simulink model "SF023A_TunSelnAuthy"  (R2013b)
settings: Solver=FixedStepDiscrete  SolverMode=SingleTasking  StartTime=0.0  StopTime=1  FixedStep=0.002  RelTol=1e-3
values from neighbouring files (symbols this model uses):
  ARCHGLBPRM_FLOATZEROTHD_ULS_F32 = DataDict.Constant    [SF023A_TunSelnAuthy_DataDict.m]
  E_NOT_OK = DataDict.Constant    [SF023A_TunSelnAuthy_DataDict.m]
  E_OK = DataDict.Constant    [SF023A_TunSelnAuthy_DataDict.m]
  TUNSELNAUTHY_XCPVEHSPDTHD_KPH_F32 = DataDict.ConfigParam    [SF023A_TunSelnAuthy_DataDict.m]
  TunSelnAuthyTunSelnRtDiCmd = DataDict.Calibration    [SF023A_TunSelnAuthy_DataDict.m]
libraries: simulink x3, FixdToFloat x2, LnrIntrpn x2, FloatToFixd x1
settings Model: Creator=TZ5743  LastModifiedBy=DZ1YRM
settings SolverCC: AutoInsertRateTranBlk=on  InsertRTBMode=Always
settings DataIOCC: LimitDataPoints=off  SaveFormat=Structure  ReturnWorkspaceOutputs=on
settings OptimizationCC: BlockReduction=off  InlineParams=on  ZeroExternalMemoryAtStartup=off  ZeroInternalMemoryAtStartup=off  OptimizeModelRefInitCode=on  LifeSpan=1
settings DebuggingCC: SignalInfNanChecking=error  SignalRangeChecking=warning  UnderspecifiedInitializationDetection=Simplified  SolverPrmCheckMsg=error  InheritedTsInSrcMsg=error  DiscreteInheritContinuousMsg=error  SingleTaskRateTransMsg=error  TasksWithSamePriorityMsg=error  SigSpecEnsureSampleTimeMsg=error  CheckMatrixSingularityMsg=error  ParameterUnderflowMsg=error  ParameterPrecisionLossMsg=error  ParameterTunabilityLossMsg=error  FixptConstUnderflowMsg=warning  FixptConstOverflowMsg=warning  VectorMatrixConversionMsg=error  SignalLabelMismatchMsg=error  UnconnectedInputMsg=error  UnconnectedOutputMsg=error  UnconnectedLineMsg=error  SFcnCompatibilityMsg=error  UniqueDataStoreMsg=warning  BusObjectLabelMismatch=error  RootOutportRequireBusObject=error  AssertControl=DisableAll  ModelReferenceIOMsg=error  ModelReferenceVersionMismatchMessage=warning  ModelReferenceIOMismatchMessage=error  ModelReferenceCSMismatchMessage=warning  ModelReferenceDataLoggingMessage=error  StateNameClashWarn=warning  StrictBusMsg=ErrorOnBusTreatedAsVector  NonBusSignalsTreatedAsBus=error  SFUnexpectedBacktrackingDiag=error  SFInvalidInputDataAccessInChartInitDiag=error  SFNoUnconditionalDefaultTransitionDiag=error  SFTransitionOutsideNaturalParentDiag=error  SFUnconditionalTransitionShadowingDiag=error  SFUndirectedBroadcastEventsDiag=error
settings ModelReferenceCC: ModelReferenceNumInstancesAllowed=Single
settings RTWCC: SystemTargetFile=autosar.tlc  GenCodeOnly=on  TemplateMakefile=ert_default_tmf  Description=AUTOSAR  GenerateReport=on  ProcessScript=autosar_make_rtw_hook  LaunchReport=on
settings CodeAppCC: GenerateComments=off  IgnoreCustomStorageClasses=off  CustomSymbolStrType=$N$R$M  CustomSymbolStrBlkIO=$N$M  SimulinkBlockComments=off
settings STFCustomTargetCC: ParMdlRefBuildCompliant=on  CompOptLevelCompliant=on  IncludeMdlTerminateFcn=off  CombineOutputUpdateFcns=on  SuppressErrorStatus=on  ERTFirstTimeCompliant=on  ERTCustomFileBanners=on  SupportNonFinite=off  SupportComplex=off  SupportContinuousTime=off  SupportNonInlinedSFcns=off  MATLABClassNameForMDSCustomization=Simulink.SoftwareTarget.ERTCustomization  AutosarCompliant=on  GRTInterface=off  SystemTargetFile=autosar.tlc
settings ERTTargetCC: CodeReplacementLibrary=ANSI_C  ConcurrentExecutionCompliant=off  IncludeMdlTerminateFcn=off  SuppressErrorStatus=on  SupportNonFinite=off  SupportComplex=off  ModelStepFunctionPrototypeControlCompliant=off  CPPClassGenCompliant=off  AutosarCompliant=on  InlinedParameterPlacement=NonHierarchical  ERTCustomFileTemplate=example_file_process.tlc  EnableUserReplacementTypes=on

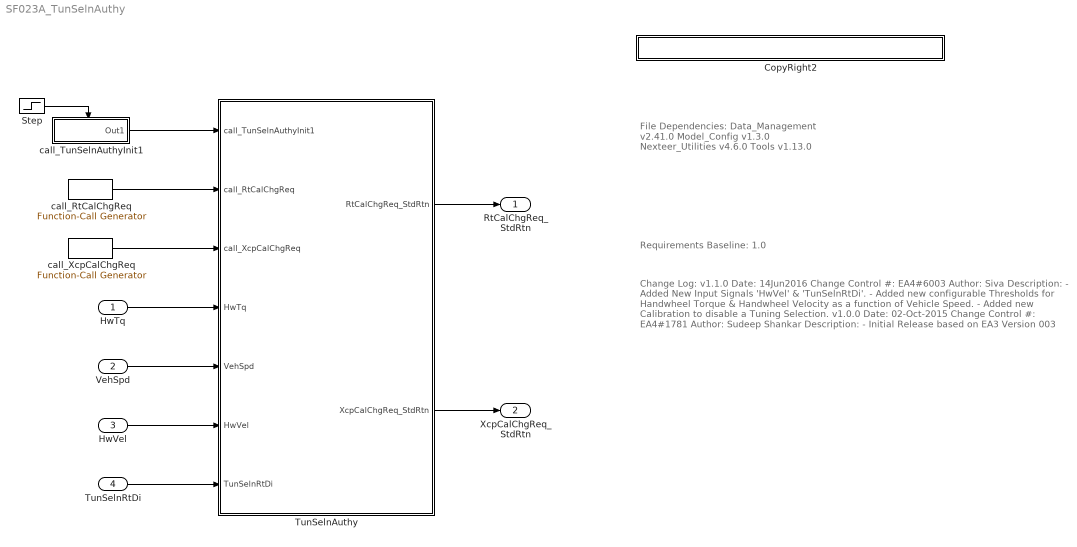
== system SF023A_TunSelnAuthy ==
  note: File Dependencies:
      |
      | Data_Management v2.41.0
      | Model_Config v1.3.0
      | Nexteer_Utilities v4.6.0
      | Tools v1.13.0
  note: Requirements Baseline: 1.0
  note: Change Log:
      |
      | v1.1.0
      | Date: 14Jun2016
      | Change Control #: EA4#6003
      | Author: Siva
      | Description:
      | - Added New Input Signals 'HwVel' & 'TunSelnRtDi'.
      | - Added new configurable Thresholds for Handwheel
      |   Torque & Handwheel Velocity as a function of Vehicle Speed.
      | - Added new Calibration to disable a Tuning Selection.
      |
      |
      |
      | v1.0.0
      | Date: 02-Oct-2015
      | Change Control #: EA4#1781
      | Author:  Sudeep Shankar
      | Description:
      | - Initial Release based on EA3 Version 003
  HwTq : Inport
  VehSpd : Inport  Port=2
  HwVel : Inport  Port=3
  TunSelnRtDi : Inport  Port=4
  CopyRight2 : Subsystem  Description=|  mask(Copyright Information){none=on}
      | Copyright info block.                                               
      |                                                                     
      | Place copyright information at the top of every subsystem in design.
      mask prompts: none "No parameters"
      mask help: Place copyright information at the top of every subsystem in design.
      mask Display:
      | NxtrConf = 'Nexteer Confidential';
      | 
      | sys = bdroot; %handle for the current model ("system")
      | first = get_param(sys,'Created');
      | if(isempty(first))
      |     first = datestr(now,'yyyy');
      | else
      |     first = first(end-3:end);  %year is last four digits
      | end
      | 
      | last = get_param(sys,'LastModifiedDate');
      | if isempty(last)
      |     last = datestr(now,'yyyy');
      | else
      |     last = last(end-3:end);
      | end
      | 
      | if strcmp(first,last)
      |     fprintf('%s -- Copyright %s Nexteer',NxtrConf,first)
      | else
      |     fprintf('%s -- %s%s- %s Nexteer',NxtrConf,char(169),first,last)
      | end
  Step : Step  Time=.001  Before=1  After=0  SampleTime=0
  TunSelnAuthy : Subsystem
  call_RtCalChgReq : simulink/Ports & Subsystems/Function-Call Generator  RequirementInfo={} %GIDa_4433d5fa_0132_44b0_b84d_e939d42c366f  sample_time=0.002  numberOfIterations=1
  call_TunSelnAuthyInit1 : Subsystem  TreatAsAtomicUnit=on
  call_XcpCalChgReq : simulink/Ports & Subsystems/Function-Call Generator  RequirementInfo={} %GIDa_23fa016c_8166_4aea_8e32_dd1f72dbacf0  sample_time=0.002  numberOfIterations=1
  RtCalChgReq_StdRtn : Outport
  XcpCalChgReq_StdRtn : Outport  Port=2
  wires:
  VehSpd/1 -> TunSelnAuthy/5(VehSpd)
  HwTq/1 -> TunSelnAuthy/4(HwTq)
  TunSelnAuthy/1(RtCalChgReq_StdRtn) -> RtCalChgReq_StdRtn/1
  TunSelnAuthy/2(XcpCalChgReq_StdRtn) -> XcpCalChgReq_StdRtn/1
  call_TunSelnAuthyInit1/1(Out1) -> TunSelnAuthy/1(call_TunSelnAuthyInit1)
  Step/1 -> call_TunSelnAuthyInit1/Enable
  call_RtCalChgReq/1 -> TunSelnAuthy/2(call_RtCalChgReq)
  call_XcpCalChgReq/1 -> TunSelnAuthy/3(call_XcpCalChgReq)
  TunSelnRtDi/1 -> TunSelnAuthy/7(TunSelnRtDi)
  HwVel/1 -> TunSelnAuthy/6(HwVel)

== system SF023A_TunSelnAuthy/CopyRight2 ==

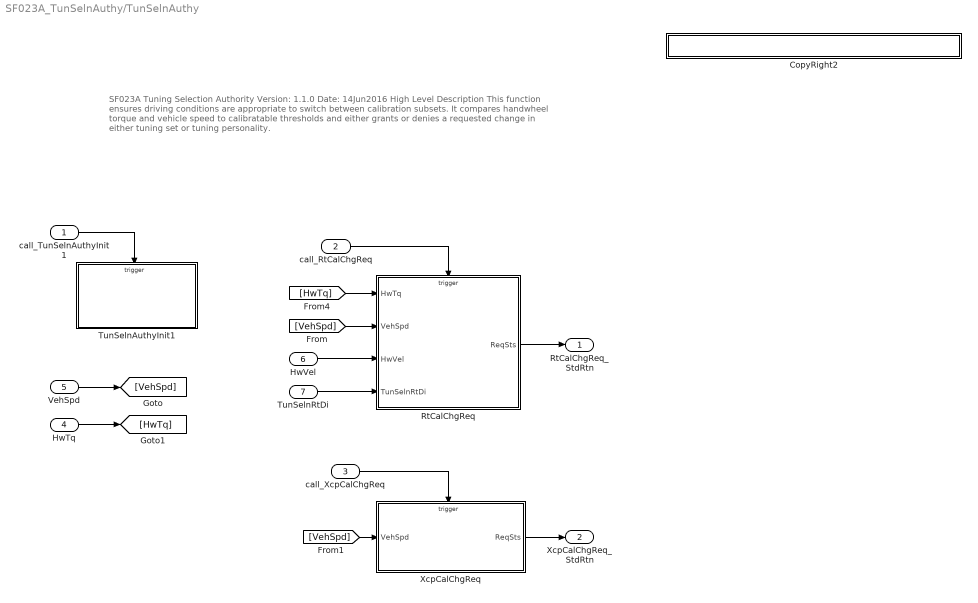
== system SF023A_TunSelnAuthy/TunSelnAuthy ==
  note: SF023A Tuning Selection Authority
      | Version: 1.1.0
      | Date: 14Jun2016
      |
      |
      |  High Level Description
      |      This function ensures driving conditions are appropriate to switch between calibration subsets.
      |      It compares handwheel torque and vehicle speed to calibratable thresholds and either grants or
      |     denies a requested change in either tuning set or tuning personality.
  call_TunSelnAuthyInit1 : Inport
  call_RtCalChgReq : Inport  Port=2
  call_XcpCalChgReq : Inport  Port=3
  HwTq : Inport  RequirementInfo="{'linktype_rmi_doors' '0000a54f (/E-STEER Core/SubSystem Specifications/Application Functions/SF023A Tuning Select Authority)' '#SF023A_9' 'true' 'REQ:  SF023A_9' '' } %GIDa_2361467c_0a1e_49a3_921d_c52f078b4324"  Port=4
  VehSpd : Inport  RequirementInfo="{'linktype_rmi_doors' '0000a54f (/E-STEER Core/SubSystem Specifications/Application Functions/SF023A Tuning Select Authority)' '#SF023A_33' 'true' 'REQ:  SF023A_33' '' } %GIDa_545f52df_7867_44c0_abd6_0d63db08a9af"  Port=5
  HwVel : Inport  RequirementInfo="{'linktype_rmi_doors' '0000a54f (/E-STEER Core/SubSystem Specifications/Application Functions/SF023A Tuning Select Authority)' '#SF023A_61' 'true' 'REQ:  SF023A_61' '' } %GIDa_db597ef0_52f4_4914_83fd_2cee657730d8"  Port=6
  TunSelnRtDi : Inport  RequirementInfo="{'linktype_rmi_doors' '0000a54f (/E-STEER Core/SubSystem Specifications/Application Functions/SF023A Tuning Select Authority)' '#SF023A_55' 'true' 'REQ:  SF023A_55' '' } %GIDa_ed13b7ea_2e8c_410a_9649_d0a9884dc505"  Port=7
  CopyRight2 : Subsystem  Description=|  mask(Copyright Information){none=on}
      | Copyright info block.                                               
      |                                                                     
      | Place copyright information at the top of every subsystem in design.
      mask prompts: none "No parameters"
      mask help: Place copyright information at the top of every subsystem in design.
      mask Display:
      | NxtrConf = 'Nexteer Confidential';
      | 
      | sys = bdroot; %handle for the current model ("system")
      | first = get_param(sys,'Created');
      | if(isempty(first))
      |     first = datestr(now,'yyyy');
      | else
      |     first = first(end-3:end);  %year is last four digits
      | end
      | 
      | last = get_param(sys,'LastModifiedDate');
      | if isempty(last)
      |     last = datestr(now,'yyyy');
      | else
      |     last = last(end-3:end);
      | end
      | 
      | if strcmp(first,last)
      |     fprintf('%s -- Copyright %s Nexteer',NxtrConf,first)
      | else
      |     fprintf('%s -- %s%s- %s Nexteer',NxtrConf,char(169),first,last)
      | end
  RtCalChgReq : Subsystem  TreatAsAtomicUnit=on
  TunSelnAuthyInit1 : Subsystem  TreatAsAtomicUnit=on
  XcpCalChgReq : Subsystem  TreatAsAtomicUnit=on
  RtCalChgReq_StdRtn : Outport  RequirementInfo="{'linktype_rmi_doors' '0000a54f (/E-STEER Core/SubSystem Specifications/Application Functions/SF023A Tuning Select Authority)' '#SF023A_46' 'true' 'REQ:  SF023A_46' '' } %GIDa_5ae6f0da_7471_4865_86ef_e3dddede8f8a"
  XcpCalChgReq_StdRtn : Outport  RequirementInfo="{'linktype_rmi_doors' '0000a54f (/E-STEER Core/SubSystem Specifications/Application Functions/SF023A Tuning Select Authority)' '#SF023A_47' 'true' 'REQ:  SF023A_47' '' } %GIDa_16ee282d_676f_45f0_a05f_c95169e43b19"  Port=2
  wires:
  call_TunSelnAuthyInit1/1 -> TunSelnAuthyInit1/Trigger
  call_XcpCalChgReq/1 -> XcpCalChgReq/Trigger
  [VehSpd] -> RtCalChgReq/2(VehSpd)
  call_RtCalChgReq/1 -> RtCalChgReq/Trigger
  [HwTq] -> RtCalChgReq/1(HwTq)
  RtCalChgReq/1(ReqSts) -> RtCalChgReq_StdRtn/1
  [VehSpd] -> XcpCalChgReq/1(VehSpd)
  XcpCalChgReq/1(ReqSts) -> XcpCalChgReq_StdRtn/1
  VehSpd/1 -> [VehSpd]
  HwTq/1 -> [HwTq]
  TunSelnRtDi/1 -> RtCalChgReq/4(TunSelnRtDi)
  HwVel/1 -> RtCalChgReq/3(HwVel)

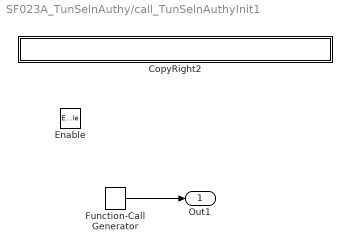
== system SF023A_TunSelnAuthy/call_TunSelnAuthyInit1 ==
  Enable : EnablePort
  CopyRight2 : Subsystem  Description=|  mask(Copyright Information){none=on}
      | Copyright info block.                                               
      |                                                                     
      | Place copyright information at the top of every subsystem in design.
      mask prompts: none "No parameters"
      mask help: Place copyright information at the top of every subsystem in design.
      mask Display:
      | NxtrConf = 'Nexteer Confidential';
      | 
      | sys = bdroot; %handle for the current model ("system")
      | first = get_param(sys,'Created');
      | if(isempty(first))
      |     first = datestr(now,'yyyy');
      | else
      |     first = first(end-3:end);  %year is last four digits
      | end
      | 
      | last = get_param(sys,'LastModifiedDate');
      | if isempty(last)
      |     last = datestr(now,'yyyy');
      | else
      |     last = last(end-3:end);
      | end
      | 
      | if strcmp(first,last)
      |     fprintf('%s -- Copyright %s Nexteer',NxtrConf,first)
      | else
      |     fprintf('%s -- %s%s- %s Nexteer',NxtrConf,char(169),first,last)
      | end
  Function-Call Generator : simulink/Ports & Subsystems/Function-Call Generator  sample_time=.002  numberOfIterations=1
  Out1 : Outport
  wires:
  Function-Call Generator/1 -> Out1/1

== system SF023A_TunSelnAuthy/TunSelnAuthy/CopyRight2 ==

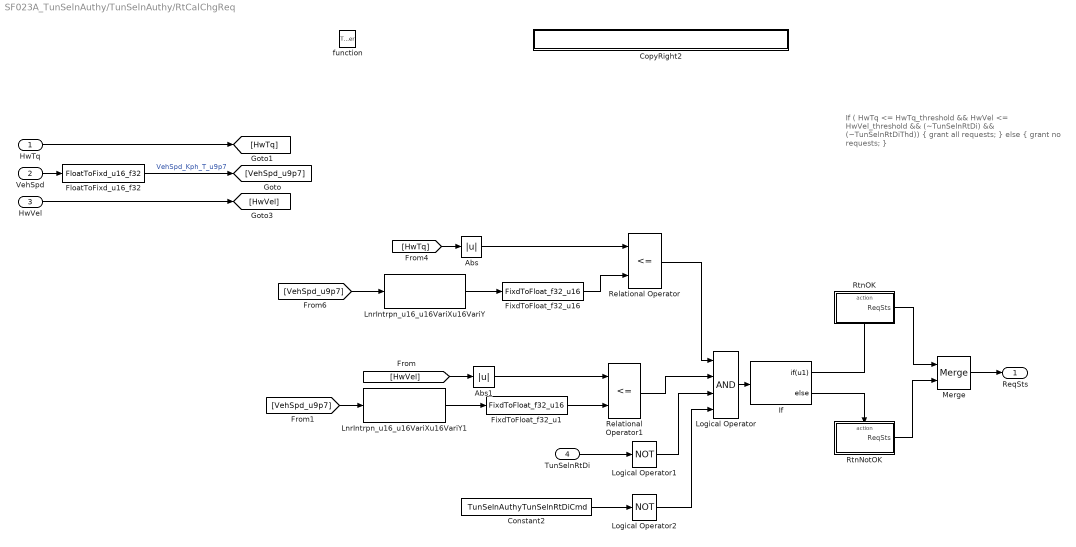
== system SF023A_TunSelnAuthy/TunSelnAuthy/RtCalChgReq ==
  note: If ( HwTq <= HwTq_threshold &&
      |      HwVel <= HwVel_threshold
      |    && (~TunSelnRtDi) && (~TunSelnRtDiThd))
      | {
      |  grant all requests;
      | }
      | else
      | {
      |  grant no requests;
      | }
  HwTq : Inport
  VehSpd : Inport  Port=2
  HwVel : Inport  Port=3
  TunSelnRtDi : Inport  RequirementInfo="{'linktype_rmi_doors' '0000a54f (/E-STEER Core/SubSystem Specifications/Application Functions/SF023A Tuning Select Authority)' '#SF023A_56' 'true' 'REQ:  SF023A_56' '' } %GIDa_0206bc00_0a03_4ad4_a51f_c7292f2e9242"  Port=4
  function : TriggerPort  TriggerType=function-call
  Abs : Abs
  Abs1 : Abs
  Constant2 : Constant  RequirementInfo="{'linktype_rmi_doors' '0000a54f (/E-STEER Core/SubSystem Specifications/Application Functions/SF023A Tuning Select Authority)' '#SF023A_56' 'true' 'REQ:  SF023A_56' '' } %GIDa_81482e17_2f66_4bcb_bed5_dbc1e0810ef7"  Value=TunSelnAuthyTunSelnRtDiCmd
  CopyRight2 : Subsystem  Description=|  mask(Copyright Information){none=on}
      | Copyright info block.                                               
      |                                                                     
      | Place copyright information at the top of every subsystem in design.
      mask prompts: none "No parameters"
      mask help: Place copyright information at the top of every subsystem in design.
      mask Display:
      | NxtrConf = 'Nexteer Confidential';
      | 
      | sys = bdroot; %handle for the current model ("system")
      | first = get_param(sys,'Created');
      | if(isempty(first))
      |     first = datestr(now,'yyyy');
      | else
      |     first = first(end-3:end);  %year is last four digits
      | end
      | 
      | last = get_param(sys,'LastModifiedDate');
      | if isempty(last)
      |     last = datestr(now,'yyyy');
      | else
      |     last = last(end-3:end);
      | end
      | 
      | if strcmp(first,last)
      |     fprintf('%s -- Copyright %s Nexteer',NxtrConf,first)
      | else
      |     fprintf('%s -- %s%s- %s Nexteer',NxtrConf,char(169),first,last)
      | end
  FixdToFloat_f32_u1 : FixdToFloat/FixdToFloat_f32_u16  Param1=10
  FixdToFloat_f32_u16 : FixdToFloat/FixdToFloat_f32_u16  Param1=12
  FloatToFixd_u16_f32 : FloatToFixd/FloatToFixd_u16_f32  Param1=7
  If : If  IfExpression=u1
  LnrIntrpn_u16_u16VariXu16VariY : LnrIntrpn/LnrIntrpn_u16_u16VariXu16VariY  RequirementInfo="{'linktype_rmi_doors' '0000a54f (/E-STEER Core/SubSystem Specifications/Application Functions/SF023A Tuning Select Authority)' '#SF023A_60' 'true' 'REQ:  SF023A_60' '' } %GIDa_aa00006d_b0c1_468f_860b_ccc5f3ecd591"  XTbl=TunSelnAuthyVehSpdX  YTbl=TunSelnAuthyHwTqY
      settings: AttributesFormatString=Lnr ( u16VariX , u16VariY )
  LnrIntrpn_u16_u16VariXu16VariY1 : LnrIntrpn/LnrIntrpn_u16_u16VariXu16VariY  RequirementInfo="{'linktype_rmi_doors' '0000a54f (/E-STEER Core/SubSystem Specifications/Application Functions/SF023A Tuning Select Authority)' '#SF023A_59' 'true' 'REQ:  SF023A_59' '' } %GIDa_6ca16c24_d5ab_4d95_898b_4104d29d42f3"  XTbl=TunSelnAuthyVehSpdX  YTbl=TunSelnAuthyHwVelY
      settings: AttributesFormatString=Lnr ( u16VariX , u16VariY )
  Logical Operator : Logic  Inputs=4  AllPortsSameDT=off  OutDataTypeStr=boolean
  Logical Operator1 : Logic  RequirementInfo="{'linktype_rmi_doors' '0000a54f (/E-STEER Core/SubSystem Specifications/Application Functions/SF023A Tuning Select Authority)' '#SF023A_56' 'true' 'REQ:  SF023A_56' '' } %GIDa_59c93d5c_08e6_4b57_969c_8230f6851426"  Operator=NOT  AllPortsSameDT=off  OutDataTypeStr=boolean
  Logical Operator2 : Logic  RequirementInfo="{'linktype_rmi_doors' '0000a54f (/E-STEER Core/SubSystem Specifications/Application Functions/SF023A Tuning Select Authority)' '#SF023A_56' 'true' 'REQ:  SF023A_56' '' } %GIDa_f65f11cf_1a83_4b4c_8f94_bf0a1c84dc81"  Operator=NOT  AllPortsSameDT=off  OutDataTypeStr=boolean
  Merge : Merge
  Relational Operator : RelationalOperator  RequirementInfo="{'linktype_rmi_doors' '0000a54f (/E-STEER Core/SubSystem Specifications/Application Functions/SF023A Tuning Select Authority)' '#SF023A_48' 'true' 'REQ:  SF023A_48' '' } %GIDa_ed988791_d00b_462e_a6ff_ecd481b56755"  Operator=<=  OutDataTypeStr=boolean
  Relational Operator1 : RelationalOperator  RequirementInfo="{'linktype_rmi_doors' '0000a54f (/E-STEER Core/SubSystem Specifications/Application Functions/SF023A Tuning Select Authority)' '#SF023A_48' 'true' 'REQ:  SF023A_48' '' } %GIDa_53b8fd5a_ad56_4a74_b7c9_2c6022f47223"  Operator=<=  OutDataTypeStr=boolean
  RtnNotOK : Subsystem  TreatAsAtomicUnit=on
  RtnOK : Subsystem  TreatAsAtomicUnit=on
  ReqSts : Outport
  wires:
  LnrIntrpn_u16_u16VariXu16VariY1/1 -> FixdToFloat_f32_u1/1
  If/1 -> RtnOK/Action
  If/2 -> RtnNotOK/Action
  Merge/1 -> ReqSts/1
  RtnOK/1(ReqSts) -> Merge/1
  RtnNotOK/1(ReqSts) -> Merge/2
  [HwTq] -> Abs/1
  Relational Operator1/1 -> Logical Operator/2
  Relational Operator/1 -> Logical Operator/1
  Constant2/1 -> Logical Operator2/1
  Logical Operator/1 -> If/1
  TunSelnRtDi/1 -> Logical Operator1/1
  VehSpd/1 -> FloatToFixd_u16_f32/1
  HwTq/1 -> [HwTq]
  HwVel/1 -> [HwVel]
  Logical Operator1/1 -> Logical Operator/3
  [VehSpd_u9p7] -> LnrIntrpn_u16_u16VariXu16VariY/1
  Logical Operator2/1 -> Logical Operator/4
  [VehSpd_u9p7] -> LnrIntrpn_u16_u16VariXu16VariY1/1
  [HwVel] -> Abs1/1
  Abs/1 -> Relational Operator/1
  LnrIntrpn_u16_u16VariXu16VariY/1 -> FixdToFloat_f32_u16/1
  Abs1/1 -> Relational Operator1/1
  FloatToFixd_u16_f32/1 -> [VehSpd_u9p7]  "VehSpd_Kph_T_u9p7"
  FixdToFloat_f32_u1/1 -> Relational Operator1/2
  FixdToFloat_f32_u16/1 -> Relational Operator/2

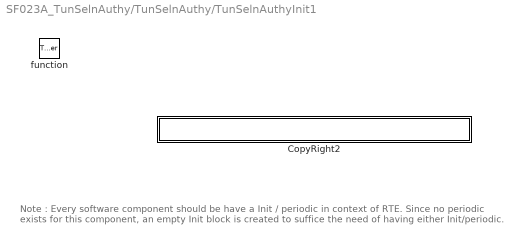
== system SF023A_TunSelnAuthy/TunSelnAuthy/TunSelnAuthyInit1 ==
  note: Note : Every software component should be have a Init / periodic in context of RTE. Since no periodic exists for this component, an empty
      | Init block is created to suffice the need of having either Init/periodic.
  function : TriggerPort  TriggerType=function-call
  CopyRight2 : Subsystem  Description=|  mask(Copyright Information){none=on}
      | Copyright info block.                                               
      |                                                                     
      | Place copyright information at the top of every subsystem in design.
      mask prompts: none "No parameters"
      mask help: Place copyright information at the top of every subsystem in design.
      mask Display:
      | NxtrConf = 'Nexteer Confidential';
      | 
      | sys = bdroot; %handle for the current model ("system")
      | first = get_param(sys,'Created');
      | if(isempty(first))
      |     first = datestr(now,'yyyy');
      | else
      |     first = first(end-3:end);  %year is last four digits
      | end
      | 
      | last = get_param(sys,'LastModifiedDate');
      | if isempty(last)
      |     last = datestr(now,'yyyy');
      | else
      |     last = last(end-3:end);
      | end
      | 
      | if strcmp(first,last)
      |     fprintf('%s -- Copyright %s Nexteer',NxtrConf,first)
      | else
      |     fprintf('%s -- %s%s- %s Nexteer',NxtrConf,char(169),first,last)
      | end

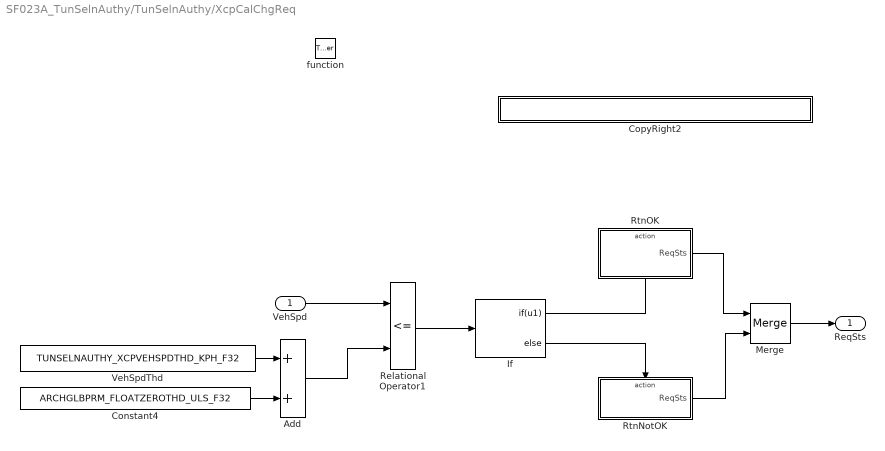
== system SF023A_TunSelnAuthy/TunSelnAuthy/XcpCalChgReq ==
  VehSpd : Inport
  function : TriggerPort  TriggerType=function-call
  Add : Sum
  Constant4 : Constant  Value=ARCHGLBPRM_FLOATZEROTHD_ULS_F32
  CopyRight2 : Subsystem  Description=|  mask(Copyright Information){none=on}
      | Copyright info block.                                               
      |                                                                     
      | Place copyright information at the top of every subsystem in design.
      mask prompts: none "No parameters"
      mask help: Place copyright information at the top of every subsystem in design.
      mask Display:
      | NxtrConf = 'Nexteer Confidential';
      | 
      | sys = bdroot; %handle for the current model ("system")
      | first = get_param(sys,'Created');
      | if(isempty(first))
      |     first = datestr(now,'yyyy');
      | else
      |     first = first(end-3:end);  %year is last four digits
      | end
      | 
      | last = get_param(sys,'LastModifiedDate');
      | if isempty(last)
      |     last = datestr(now,'yyyy');
      | else
      |     last = last(end-3:end);
      | end
      | 
      | if strcmp(first,last)
      |     fprintf('%s -- Copyright %s Nexteer',NxtrConf,first)
      | else
      |     fprintf('%s -- %s%s- %s Nexteer',NxtrConf,char(169),first,last)
      | end
  If : If  IfExpression=u1
  Merge : Merge
  Relational Operator1 : RelationalOperator  RequirementInfo="{'linktype_rmi_doors' '0000a54f (/E-STEER Core/SubSystem Specifications/Application Functions/SF023A Tuning Select Authority)' '#SF023A_49' 'true' 'REQ:  SF023A_49' '' } %GIDa_3ba4f68b_34aa_4153_92de_b26e7192a731"  Operator=<=  OutDataTypeStr=boolean
  RtnNotOK : Subsystem  TreatAsAtomicUnit=on
  RtnOK : Subsystem  TreatAsAtomicUnit=on
  VehSpdThd : Constant  Value=TUNSELNAUTHY_XCPVEHSPDTHD_KPH_F32
  ReqSts : Outport
  wires:
  Relational Operator1/1 -> If/1
  If/1 -> RtnOK/Action
  If/2 -> RtnNotOK/Action
  Merge/1 -> ReqSts/1
  RtnOK/1(ReqSts) -> Merge/1
  RtnNotOK/1(ReqSts) -> Merge/2
  VehSpdThd/1 -> Add/1
  Add/1 -> Relational Operator1/2
  Constant4/1 -> Add/2
  VehSpd/1 -> Relational Operator1/1

== system SF023A_TunSelnAuthy/call_TunSelnAuthyInit1/CopyRight2 ==

== system SF023A_TunSelnAuthy/TunSelnAuthy/RtCalChgReq/CopyRight2 ==

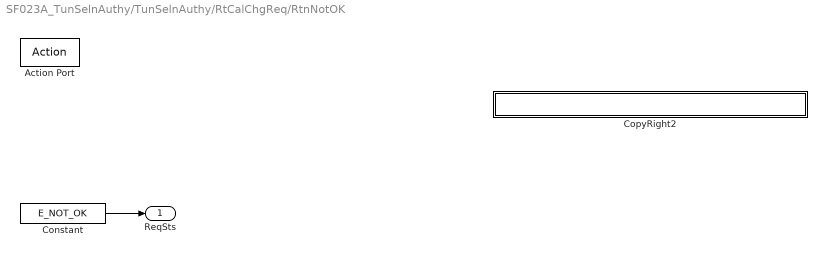
== system SF023A_TunSelnAuthy/TunSelnAuthy/RtCalChgReq/RtnNotOK ==
  Action Port : ActionPort  ActionType=else
  Constant : Constant  Value=E_NOT_OK
  CopyRight2 : Subsystem  Description=|  mask(Copyright Information){none=on}
      | Copyright info block.                                               
      |                                                                     
      | Place copyright information at the top of every subsystem in design.
      mask prompts: none "No parameters"
      mask help: Place copyright information at the top of every subsystem in design.
      mask Display:
      | NxtrConf = 'Nexteer Confidential';
      | 
      | sys = bdroot; %handle for the current model ("system")
      | first = get_param(sys,'Created');
      | if(isempty(first))
      |     first = datestr(now,'yyyy');
      | else
      |     first = first(end-3:end);  %year is last four digits
      | end
      | 
      | last = get_param(sys,'LastModifiedDate');
      | if isempty(last)
      |     last = datestr(now,'yyyy');
      | else
      |     last = last(end-3:end);
      | end
      | 
      | if strcmp(first,last)
      |     fprintf('%s -- Copyright %s Nexteer',NxtrConf,first)
      | else
      |     fprintf('%s -- %s%s- %s Nexteer',NxtrConf,char(169),first,last)
      | end
  ReqSts : Outport
  wires:
  Constant/1 -> ReqSts/1

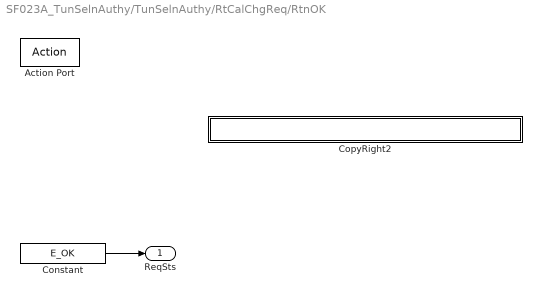
== system SF023A_TunSelnAuthy/TunSelnAuthy/RtCalChgReq/RtnOK ==
  Action Port : ActionPort  ActionType=then
  Constant : Constant  Value=E_OK
  CopyRight2 : Subsystem  Description=|  mask(Copyright Information){none=on}
      | Copyright info block.                                               
      |                                                                     
      | Place copyright information at the top of every subsystem in design.
      mask prompts: none "No parameters"
      mask help: Place copyright information at the top of every subsystem in design.
      mask Display:
      | NxtrConf = 'Nexteer Confidential';
      | 
      | sys = bdroot; %handle for the current model ("system")
      | first = get_param(sys,'Created');
      | if(isempty(first))
      |     first = datestr(now,'yyyy');
      | else
      |     first = first(end-3:end);  %year is last four digits
      | end
      | 
      | last = get_param(sys,'LastModifiedDate');
      | if isempty(last)
      |     last = datestr(now,'yyyy');
      | else
      |     last = last(end-3:end);
      | end
      | 
      | if strcmp(first,last)
      |     fprintf('%s -- Copyright %s Nexteer',NxtrConf,first)
      | else
      |     fprintf('%s -- %s%s- %s Nexteer',NxtrConf,char(169),first,last)
      | end
  ReqSts : Outport
  wires:
  Constant/1 -> ReqSts/1

== system SF023A_TunSelnAuthy/TunSelnAuthy/TunSelnAuthyInit1/CopyRight2 ==

== system SF023A_TunSelnAuthy/TunSelnAuthy/XcpCalChgReq/CopyRight2 ==

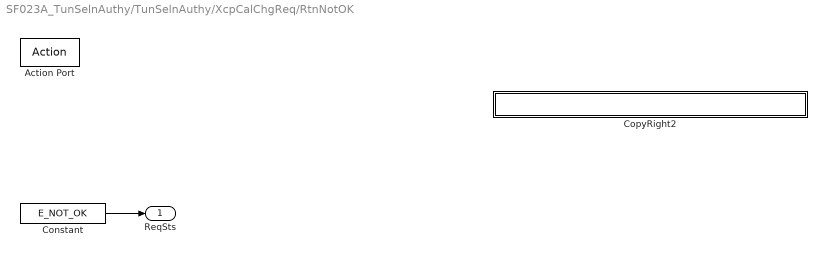
== system SF023A_TunSelnAuthy/TunSelnAuthy/XcpCalChgReq/RtnNotOK ==
  Action Port : ActionPort  ActionType=else
  Constant : Constant  Value=E_NOT_OK
  CopyRight2 : Subsystem  Description=|  mask(Copyright Information){none=on}
      | Copyright info block.                                               
      |                                                                     
      | Place copyright information at the top of every subsystem in design.
      mask prompts: none "No parameters"
      mask help: Place copyright information at the top of every subsystem in design.
      mask Display:
      | NxtrConf = 'Nexteer Confidential';
      | 
      | sys = bdroot; %handle for the current model ("system")
      | first = get_param(sys,'Created');
      | if(isempty(first))
      |     first = datestr(now,'yyyy');
      | else
      |     first = first(end-3:end);  %year is last four digits
      | end
      | 
      | last = get_param(sys,'LastModifiedDate');
      | if isempty(last)
      |     last = datestr(now,'yyyy');
      | else
      |     last = last(end-3:end);
      | end
      | 
      | if strcmp(first,last)
      |     fprintf('%s -- Copyright %s Nexteer',NxtrConf,first)
      | else
      |     fprintf('%s -- %s%s- %s Nexteer',NxtrConf,char(169),first,last)
      | end
  ReqSts : Outport
  wires:
  Constant/1 -> ReqSts/1

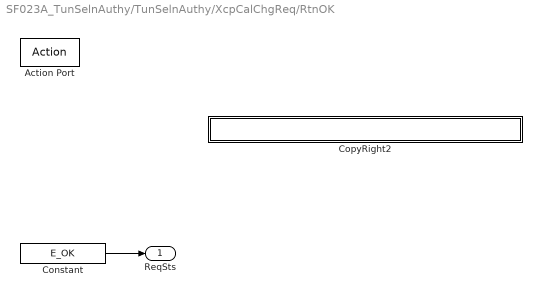
== system SF023A_TunSelnAuthy/TunSelnAuthy/XcpCalChgReq/RtnOK ==
  Action Port : ActionPort  ActionType=then
  Constant : Constant  Value=E_OK
  CopyRight2 : Subsystem  Description=|  mask(Copyright Information){none=on}
      | Copyright info block.                                               
      |                                                                     
      | Place copyright information at the top of every subsystem in design.
      mask prompts: none "No parameters"
      mask help: Place copyright information at the top of every subsystem in design.
      mask Display:
      | NxtrConf = 'Nexteer Confidential';
      | 
      | sys = bdroot; %handle for the current model ("system")
      | first = get_param(sys,'Created');
      | if(isempty(first))
      |     first = datestr(now,'yyyy');
      | else
      |     first = first(end-3:end);  %year is last four digits
      | end
      | 
      | last = get_param(sys,'LastModifiedDate');
      | if isempty(last)
      |     last = datestr(now,'yyyy');
      | else
      |     last = last(end-3:end);
      | end
      | 
      | if strcmp(first,last)
      |     fprintf('%s -- Copyright %s Nexteer',NxtrConf,first)
      | else
      |     fprintf('%s -- %s%s- %s Nexteer',NxtrConf,char(169),first,last)
      | end
  ReqSts : Outport
  wires:
  Constant/1 -> ReqSts/1

== system SF023A_TunSelnAuthy/TunSelnAuthy/RtCalChgReq/RtnNotOK/CopyRight2 ==

== system SF023A_TunSelnAuthy/TunSelnAuthy/RtCalChgReq/RtnOK/CopyRight2 ==

== system SF023A_TunSelnAuthy/TunSelnAuthy/XcpCalChgReq/RtnNotOK/CopyRight2 ==

== system SF023A_TunSelnAuthy/TunSelnAuthy/XcpCalChgReq/RtnOK/CopyRight2 ==
